simulink model "sampleModel931"  (R2021a)
settings: Solver=VariableStepAuto  StartTime=0.0  StopTime=10.0  RelTol=1e-3
undefined symbols (not defined in the file or in its folder): DiscIntNeverNeededParam, magnitude, Newton, Raphson
libraries: simulink x35, pid_lib x8
(part 1 of 2)
settings Model: Creator=user  LastModifiedBy=user

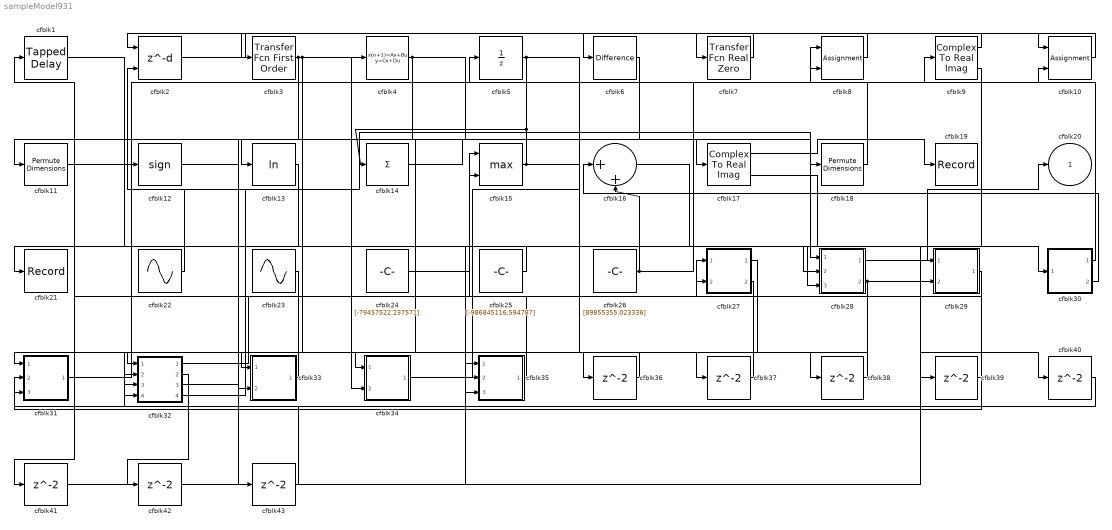
== system sampleModel931 ==
  cfblk1 : simulink/Discrete/Tapped Delay  vinit=0.0  samptime=-1  NumDelays=1  DelayOrder=Oldest  includeCurrent=off
  cfblk10 : Assignment  DiagnosticForDimensions=Warning  IndexOptions=Index vector (dialog)  Indices=1  OutputSizes=1
  cfblk11 : PermuteDimensions
  cfblk12 : Signum
  cfblk13 : Math  Operator=log  SaturateOnIntegerOverflow=on
  cfblk14 : Sum  Inputs=+
  cfblk15 : MinMax  Function=max  Inputs=2
  cfblk16 : Sum  Inputs=|++
  cfblk17 : ComplexToRealImag
  cfblk18 : PermuteDimensions
  cfblk19 : Record  FileSettingsInternal="{\"entries\":[{\"content\":{\"excelSettings\":{\"content\":{},\"type\":\"Streamout.ExcelSettings\"}},\"type\":\"Streamout.FileSettingStorage\",\"uuid\":\"344b2579-8096-44a0-829a-8fa8cea9bf3e\"}],\"packageUris\":[\"http://schema.mathworks.com/mf0/streamout_blocks/R2020a\"],\"version\":\"1.0\"}"  SignalsInternal="{\"entries\":[{\"content\":{\"signals\":[{\"content\":{\"blockPath\":[\"sampleModel931/cfblk19\"],\"channel\":[],\"dimensions\":[1],\"domain\":\"samplemodel931/cfblk19\",\"lineColor\":\"#a2142f\",\"plots\":[1],\"port\":1,\"sid\":[\"\"],\"signalID\":7177,\"signalName\":\"cfblk17:1\"},\"type\":\"RecordBlkView.Signal\",\"uuid\":\"202db960-daa0-4a0a-ad9f-c9ed2231518e\"}]},\"type\":\"RecordBlkView.InputSignals\",\"uuid\":\"c8fea5f5-595d-44bd-9296-e1420b6ba1ce\"}],\"packageUris\":[\"http://schema.mathworks.com/mf0/streamout_blocks/R2020a\"],\"version\":\"1.0\"}"  VisualizationBindings="{\"sparklinesplugin\":{\"info\":[{\"bindingParametersList\":[],\"subplotID\":1}]}}"
  cfblk2 : Delay  DelayLengthSource=Input port  SampleTime=1
      settings: InputPortMap=u0,p1
  cfblk21 : Record  FileSettingsInternal="{\"entries\":[{\"content\":{\"excelSettings\":{\"content\":{},\"type\":\"Streamout.ExcelSettings\"}},\"type\":\"Streamout.FileSettingStorage\",\"uuid\":\"47128032-d6b5-40ff-842c-bb4838ad83b6\"}],\"packageUris\":[\"http://schema.mathworks.com/mf0/streamout_blocks/R2020a\"],\"version\":\"1.0\"}"  SignalsInternal="{\"entries\":[{\"content\":{\"signals\":[{\"content\":{\"blockPath\":[\"sampleModel931/cfblk21\"],\"channel\":[],\"dimensions\":[1],\"domain\":\"samplemodel931/cfblk21\",\"lineColor\":\"#ff6929\",\"plots\":[1],\"port\":1,\"sid\":[\"\"],\"signalID\":7185,\"signalName\":\"cfblk25\"},\"type\":\"RecordBlkView.Signal\",\"uuid\":\"305fc408-6697-4ad2-987d-cf51be774916\"}]},\"type\":\"RecordBlkView.InputSignals\",\"uuid\":\"d64a9699-7d60-471f-aacd-da0b4468fcb5\"}],\"packageUris\":[\"http://schema.mathworks.com/mf0/streamout_blocks/R2020a\"],\"version\":\"1.0\"}"  VisualizationBindings="{\"sparklinesplugin\":{\"info\":[{\"bindingParametersList\":[],\"subplotID\":1}]}}"
  cfblk22 : Sin  Amplitude=[-979508255.020901]  Bias=[-315371967.281883]  SampleTime=0
  cfblk23 : Sin  Amplitude=[-6086076.617580]  Bias=[-663456107.750280]  SampleTime=0
  cfblk24 : Constant  Value=[-79457522.237571]  SampleTime=1
  cfblk25 : Constant  Value=[-986845116.594787]  SampleTime=1
  cfblk26 : Constant  Value=[89855355.023336]  SampleTime=1
  cfblk27 : Subsystem
  cfblk28 : Subsystem
  cfblk29 : Subsystem
  cfblk3 : simulink/Discrete/Transfer Fcn First Order  PoleZ=0.95  ICPrevOutput=0.0  DoSatur=off
  cfblk30 : Subsystem
  cfblk31 : Subsystem
  cfblk32 : Subsystem
  cfblk33 : Subsystem
  cfblk34 : Subsystem
  cfblk35 : Subsystem
  cfblk{36..43} (8 alike) : Delay  SampleTime=1
  cfblk4 : DiscreteStateSpace
  cfblk5 : UnitDelay  HasFrameUpgradeWarning=on
  cfblk6 : simulink/Discrete/Difference  ICPrevInput=0.0  OutMin=[]  OutMax=[]  OutDataTypeStr=Inherit: Inherit via back propagation  OutDataType=fixdt(1, 16)  OutScaling=2^-10  DoSatur=off
  cfblk7 : simulink/Discrete/Transfer Fcn Real Zero  ZeroZ=0.75  ICPrevInput=0.0  DoSatur=off
      settings: SourceProductBaseCode=SL
  cfblk8 : Assignment  DiagnosticForDimensions=Warning  IndexOptions=Index vector (dialog)  Indices=1  OutputSizes=1
  cfblk9 : ComplexToRealImag
  cfblk20 : Outport
  wires:
  cfblk2/1 -> cfblk10/1
  cfblk3/1 -> cfblk33/1(cfblk1), cfblk36/1, cfblk33/2(cfblk12)
  cfblk32/1(cfblk2) -> cfblk27/1(cfblk1)
  cfblk28/1(cfblk2) -> cfblk20/1
  cfblk35/1(cfblk2) -> cfblk15/1
  cfblk14/1 -> cfblk17/1
  cfblk11/1 -> cfblk28/1(cfblk1)
  cfblk5/1 -> cfblk14/1, cfblk34/1(cfblk1), cfblk28/3(cfblk14)
  cfblk4/1 -> cfblk11/1, cfblk18/1
  cfblk6/1 -> cfblk13/1
  cfblk8/1 -> cfblk2/1
  cfblk17/1 -> cfblk19/1
  cfblk25/1 -> cfblk21/1
  cfblk16/1 -> cfblk28/2(cfblk13)
  cfblk31/1(cfblk2) -> cfblk9/1
  cfblk33/1(cfblk2) -> cfblk32/1(cfblk1)
  cfblk18/1 -> cfblk8/1
  cfblk9/1 -> cfblk3/1
  cfblk22/1 -> cfblk2/2
  cfblk30/1(cfblk2) -> cfblk5/1
  cfblk30/2(cfblk8) -> cfblk16/1
  cfblk34/1(cfblk2) -> cfblk10/2
  cfblk29/1(cfblk2) -> cfblk31/2(cfblk13)
  cfblk32/4(cfblk16) -> cfblk4/1
  cfblk15/1 -> cfblk12/1, cfblk38/1
  cfblk24/1 -> cfblk15/2
  cfblk7/1 -> cfblk6/1
  cfblk26/1 -> cfblk8/2, cfblk16/2
  cfblk1/1 -> cfblk29/2(cfblk12)
  cfblk10/1 -> cfblk7/1
  cfblk28/2(cfblk15) -> cfblk34/2(cfblk7), cfblk40/1
  cfblk9/2 -> cfblk35/2(cfblk16)
  cfblk12/1 -> cfblk30/1(cfblk1)
  cfblk23/1 -> cfblk32/4(cfblk13)
  cfblk27/2(cfblk7) -> cfblk35/3(cfblk17)
  cfblk36/1 -> cfblk31/1(cfblk1)
  cfblk27/1(cfblk2) -> cfblk37/1
  cfblk37/1 -> cfblk1/1
  cfblk38/1 -> cfblk32/2(cfblk11)
  cfblk17/2 -> cfblk39/1
  cfblk39/1 -> cfblk27/2(cfblk6)
  cfblk40/1 -> cfblk32/3(cfblk12)
  cfblk13/1 -> cfblk41/1
  cfblk41/1 -> cfblk35/1(cfblk1)
  cfblk32/2(cfblk14) -> cfblk42/1
  cfblk42/1 -> cfblk29/1(cfblk1)
  cfblk32/3(cfblk15) -> cfblk43/1
  cfblk43/1 -> cfblk31/3(cfblk14)

== system sampleModel931/cfblk27 ==
  cfblk1 : Inport
  cfblk6 : Inport  Port=2
  cfblk3 : Constant  Value=[-684045986.620494]  SampleTime=1
  cfblk4 : Subsystem
  cfblk5 : Subsystem
  cfblk2 : Outport
  cfblk7 : Outport  Port=2
  wires:
  cfblk5/1(cfblk2) -> cfblk7/1
  cfblk6/1 -> cfblk5/1(cfblk1)
  cfblk1/1 -> cfblk5/2(cfblk13)
  cfblk3/1 -> cfblk2/1
  cfblk5/2(cfblk14) -> cfblk4/1(cfblk1)

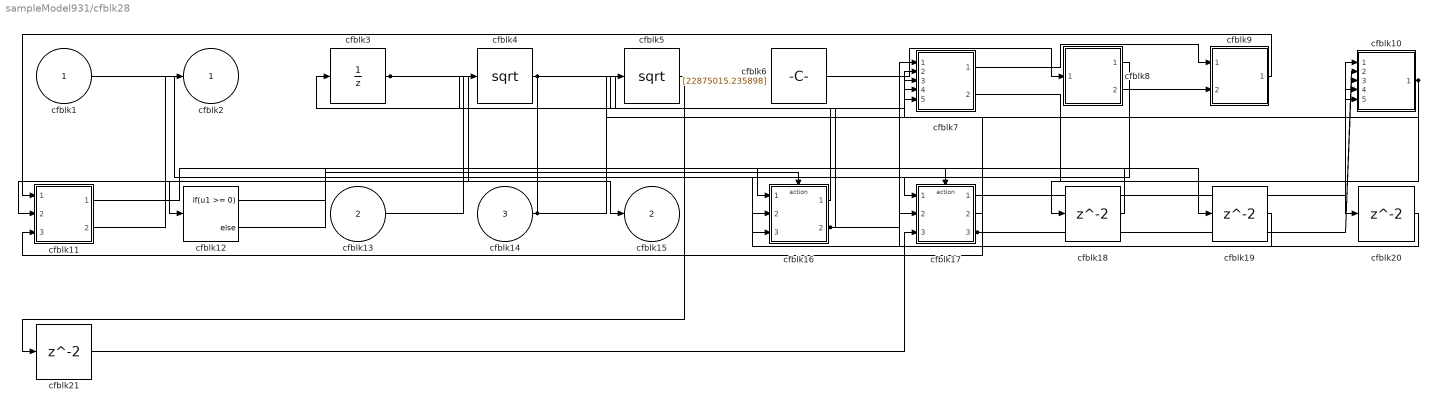
== system sampleModel931/cfblk28 ==
  cfblk1 : Inport
  cfblk13 : Inport  Port=2
  cfblk14 : Inport  Port=3
  cfblk10 : Subsystem
  cfblk11 : Subsystem
  cfblk12 : If  IfExpression=u1 >= 0  SampleTime=1
  cfblk16 : Subsystem  TreatAsAtomicUnit=on
  cfblk17 : Subsystem  TreatAsAtomicUnit=on
  cfblk{18..21} (4 alike) : Delay  SampleTime=1
  cfblk3 : UnitDelay  HasFrameUpgradeWarning=on
  cfblk4 : Sqrt  SaturateOnIntegerOverflow=on
  cfblk5 : Sqrt  SaturateOnIntegerOverflow=on
  cfblk6 : Constant  Value=[22875015.235898]  SampleTime=1
  cfblk7 : Subsystem
  cfblk8 : Subsystem
  cfblk9 : Subsystem
  cfblk2 : Outport
  cfblk15 : Outport  Port=2
  wires:
  cfblk17/1(cfblk2) -> cfblk10/1(cfblk1)
  cfblk1/1 -> cfblk17/1(cfblk1)
  cfblk7/1(cfblk2) -> cfblk9/1(cfblk1)
  cfblk10/1(cfblk2) -> cfblk7/4(cfblk12), cfblk18/1
  cfblk8/1(cfblk2) -> cfblk16/3(cfblk14)
  cfblk3/1 -> cfblk15/1, cfblk7/5(cfblk13)
  cfblk14/1 -> cfblk12/1, cfblk10/4(cfblk15)
  cfblk8/2(cfblk8) -> cfblk9/2(cfblk15)
  cfblk13/1 -> cfblk4/1
  cfblk16/1(cfblk2) -> cfblk3/1
  cfblk9/1(cfblk2) -> cfblk11/1(cfblk1)
  cfblk11/2(cfblk15) -> cfblk2/1
  cfblk4/1 -> cfblk11/2(cfblk13), cfblk7/3(cfblk11), cfblk10/5(cfblk16)
  cfblk6/1 -> cfblk8/1(cfblk1)
  cfblk16/2(cfblk15) -> cfblk7/1(cfblk1), cfblk5/1
  cfblk17/2(cfblk13) -> cfblk11/3(cfblk14)
  cfblk17/3(cfblk14) -> cfblk7/2(cfblk10), cfblk10/2(cfblk13), cfblk10/3(cfblk14)
  cfblk12/1 -> cfblk16/Action
  cfblk12/2 -> cfblk17/Action
  cfblk18/1 -> cfblk16/1(cfblk1)
  cfblk11/1(cfblk2) -> cfblk19/1
  cfblk19/1 -> cfblk17/2(cfblk11)
  cfblk7/2(cfblk14) -> cfblk20/1
  cfblk20/1 -> cfblk16/2(cfblk13)
  cfblk5/1 -> cfblk21/1
  cfblk21/1 -> cfblk17/3(cfblk12)

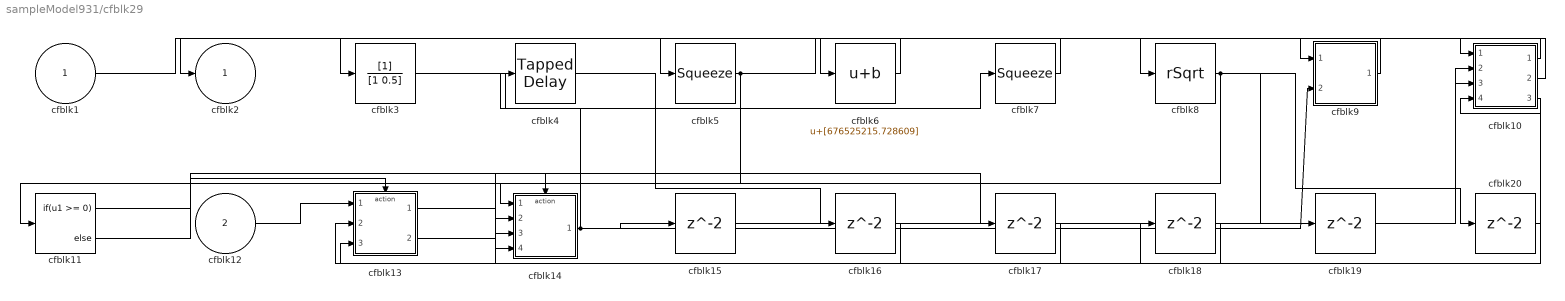
== system sampleModel931/cfblk29 ==
  cfblk1 : Inport
  cfblk12 : Inport  Port=2
  cfblk10 : Subsystem
  cfblk11 : If  IfExpression=u1 >= 0  SampleTime=1
  cfblk13 : Subsystem  TreatAsAtomicUnit=on
  cfblk14 : Subsystem  TreatAsAtomicUnit=on
  cfblk{15..20} (6 alike) : Delay  SampleTime=1
  cfblk3 : DiscreteFilter  SampleTime=1
  cfblk4 : simulink/Discrete/Tapped Delay  vinit=0.0  samptime=-1  NumDelays=1  DelayOrder=Oldest  includeCurrent=off
  cfblk5 : Squeeze
  cfblk6 : Bias  Bias=[676525215.728609]
  cfblk7 : Squeeze
  cfblk8 : Sqrt  Operator=rSqrt  AlgorithmType=Newton-Raphson  SaturateOnIntegerOverflow=on
  cfblk9 : Subsystem
  cfblk2 : Outport
  wires:
  cfblk9/1(cfblk2) -> cfblk3/1
  cfblk3/1 -> cfblk7/1
  cfblk6/1 -> cfblk2/1
  cfblk7/1 -> cfblk6/1
  cfblk12/1 -> cfblk13/1(cfblk1)
  cfblk1/1 -> cfblk5/1
  cfblk8/1 -> cfblk14/1(cfblk1), cfblk19/1, cfblk20/1
  cfblk5/1 -> cfblk10/1(cfblk1), cfblk11/1, cfblk14/4(cfblk14)
  cfblk10/1(cfblk2) -> cfblk8/1
  cfblk14/1(cfblk2) -> cfblk9/2(cfblk8), cfblk4/1, cfblk15/1
  cfblk10/2(cfblk9) -> cfblk9/1(cfblk1)
  cfblk10/3(cfblk10) -> cfblk13/3(cfblk16)
  cfblk11/1 -> cfblk13/Action
  cfblk11/2 -> cfblk14/Action
  cfblk15/1 -> cfblk10/2(cfblk6)
  cfblk4/1 -> cfblk16/1
  cfblk16/1 -> cfblk13/2(cfblk15)
  cfblk13/1(cfblk2) -> cfblk17/1
  cfblk17/1 -> cfblk14/2(cfblk12)
  cfblk13/2(cfblk17) -> cfblk18/1
  cfblk18/1 -> cfblk14/3(cfblk13)
  cfblk19/1 -> cfblk10/3(cfblk7)
  cfblk20/1 -> cfblk10/4(cfblk8)

== system sampleModel931/cfblk30 ==
  cfblk1 : Inport
  cfblk3 : DiscreteFir  SampleTime=1
  cfblk4 : DiscreteStateSpace
  cfblk5 : Product
  cfblk6 : Product
  cfblk7 : Constant  Value=[840177180.209382]  SampleTime=1
  cfblk2 : Outport
  cfblk8 : Outport  Port=2
  wires:
  cfblk7/1 -> cfblk6/1
  cfblk5/1 -> cfblk3/1, cfblk4/1
  cfblk3/1 -> cfblk6/2
  cfblk4/1 -> cfblk8/1
  cfblk1/1 -> cfblk5/1, cfblk5/2
  cfblk6/1 -> cfblk2/1

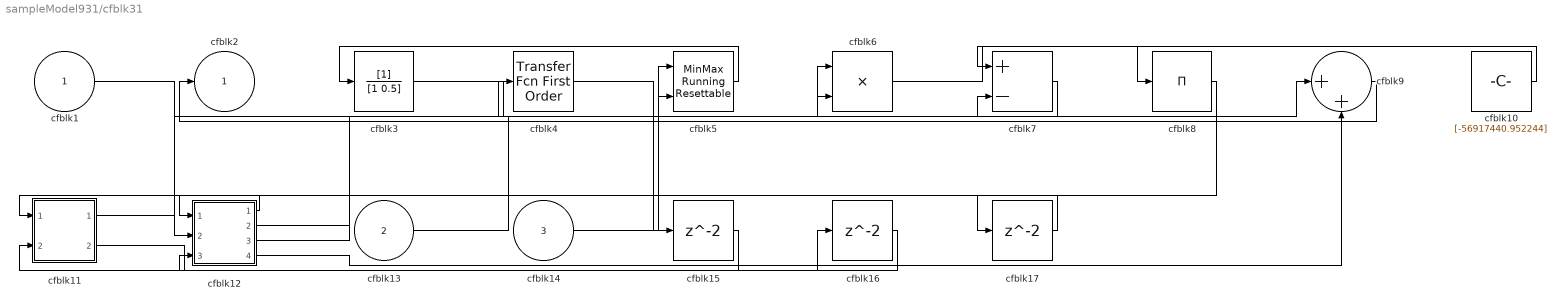
== system sampleModel931/cfblk31 ==
  cfblk1 : Inport
  cfblk13 : Inport  Port=2
  cfblk14 : Inport  Port=3
  cfblk10 : Constant  Value=[-56917440.952244]  SampleTime=1
  cfblk11 : Subsystem
  cfblk12 : Subsystem
  cfblk15 : Delay  SampleTime=1
  cfblk16 : Delay  SampleTime=1
  cfblk17 : Delay  SampleTime=1
  cfblk3 : DiscreteFilter  SampleTime=1
  cfblk4 : simulink/Discrete/Transfer Fcn First Order  PoleZ=0.95  ICPrevOutput=0.0  DoSatur=off
  cfblk5 : simulink/Math Operations/MinMax Running Resettable  Function=min  vinit=0.0
  cfblk6 : Product
  cfblk7 : Sum  Inputs=+-
  cfblk8 : Product  Inputs=*
  cfblk9 : Sum  Inputs=|++
  cfblk2 : Outport
  wires:
  cfblk6/1 -> cfblk8/1
  cfblk9/1 -> cfblk2/1
  cfblk5/1 -> cfblk3/1
  cfblk3/1 -> cfblk6/1
  cfblk10/1 -> cfblk7/1
  cfblk7/1 -> cfblk6/2
  cfblk11/1(cfblk2) -> cfblk4/1
  cfblk13/1 -> cfblk9/1
  cfblk12/1(cfblk2) -> cfblk11/1(cfblk1)
  cfblk1/1 -> cfblk12/2(cfblk10)
  cfblk12/2(cfblk12) -> cfblk7/2
  cfblk12/3(cfblk13) -> cfblk5/1
  cfblk14/1 -> cfblk5/2
  cfblk12/4(cfblk14) -> cfblk9/2
  cfblk4/1 -> cfblk15/1
  cfblk15/1 -> cfblk11/2(cfblk6)
  cfblk11/2(cfblk7) -> cfblk16/1
  cfblk16/1 -> cfblk12/3(cfblk11)
  cfblk8/1 -> cfblk17/1
  cfblk17/1 -> cfblk12/1(cfblk1)

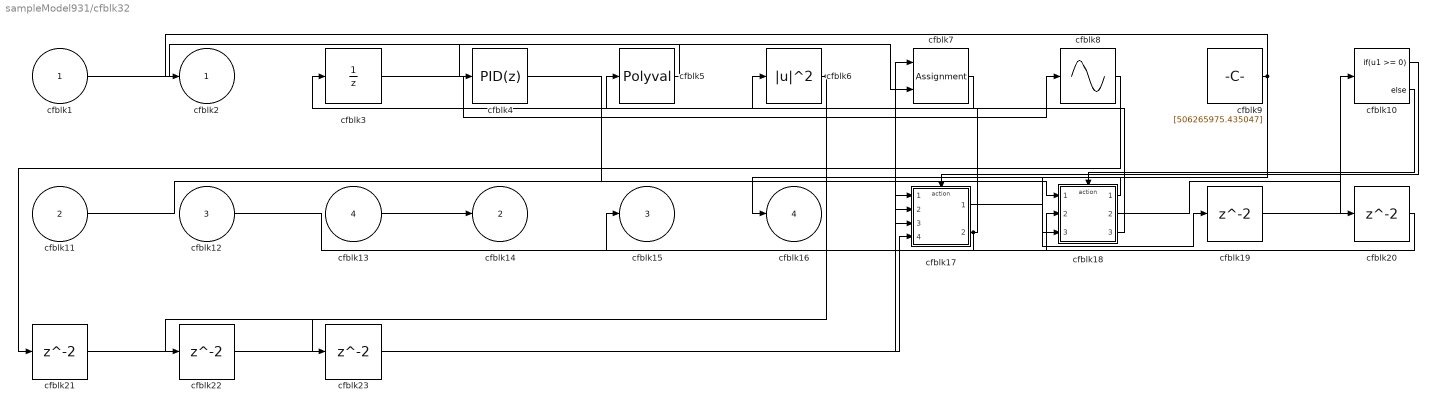
== system sampleModel931/cfblk32 ==
  cfblk1 : Inport
  cfblk11 : Inport  Port=2
  cfblk12 : Inport  Port=3
  cfblk13 : Inport  Port=4
  cfblk10 : If  IfExpression=u1 >= 0  SampleTime=1
  cfblk17 : Subsystem  TreatAsAtomicUnit=on
  cfblk18 : Subsystem  TreatAsAtomicUnit=on
  cfblk{19..23} (5 alike) : Delay  SampleTime=1
  cfblk3 : UnitDelay  HasFrameUpgradeWarning=on
  cfblk4 : pid_lib/PID Controller  Controller=PID  Form=Parallel  TimeDomain=Discrete-time  UseExternalTs=off  SampleTime=1  IntegratorMethod=Forward Euler  FilterMethod=Forward Euler  ControllerParametersSource=internal  P=1  I=1  D=0  UseFilter=on  N=100  TunerSelectOption=Transfer Function Based (PID Tuner App)  InitialConditionSource=internal  InitialConditionForIntegrator=0  InitialConditionForFilter=0  DifferentiatorICPrevScaledInput=0  ExternalReset=none  TrackingMode=off  Kt=1  LimitOutput=off  SatLimitsSource=internal  UpperSaturationLimit=inf  LowerSaturationLimit=-inf  LinearizeAsGain=off  AntiWindupMode=none  Kb=1  POutMin=[]  POutMax=[]  IOutMin=[]  IOutMax=[]  DOutMin=[]  DOutMax=[]  NOutMin=[]  NOutMax=[]  SumOutMin=[]  SumOutMax=[]  SaturationOutMin=[]  SaturationOutMax=[]  PParamMin=[]  PParamMax=[]  IParamMin=[]  IParamMax=[]  DParamMin=[]  DParamMax=[]  NParamMin=[]  NParamMax=[]  KbParamMin=[]  KbParamMax=[]  KtParamMin=[]  KtParamMax=[]  KbOutMin=[]  KbOutMax=[]  KtOutMin=[]  KtOutMax=[]  IntegratorOutMin=[]  IntegratorOutMax=[]  FilterOutMin=[]  FilterOutMax=[]  SumI1OutMin=[]  SumI1OutMax=[]  SumI2OutMin=[]  SumI2OutMax=[]  SumI3OutMin=[]  SumI3OutMax=[]  SumI4OutMin=[]  SumI4OutMax=[]  SumDOutMin=[]  SumDOutMax=[]  DifferentiatorOutMin=[]  DifferentiatorOutMax=[]  FilterDiffOutCoefMin=[]  FilterDiffOutCoefMax=[]  ReciprocalOutMin=[]  ReciprocalOutMax=[]  SumDenOutMin=[]  SumDenOutMax=[]  SumNumOutMin=[]  SumNumOutMax=[]  DivideOutMin=[]  DivideOutMax=[]  UdiffTsProdOutMin=[]  UdiffTsProdOutMax=[]  NTsProdOutMin=[]  NTsProdOutMax=[]  UintegralTsProdOutMin=[]  UintegralTsProdOutMax=[]  UngainTsProdOutMin=[]  UngainTsProdOutMax=[]  IntegratorContinuousStateAttributes=''  IntegratorStateMustResolveToSignalObject=off  IntegratorRTWStateStorageClass=Auto  FilterContinuousStateAttributes=''  FilterStateMustResolveToSignalObject=off  FilterRTWStateStorageClass=Auto  ParallelPVariant=InternalParameters  IdealPVariant=Disabled  IVariant=InternalParameters  DVariant=InternalParameters  IntegratorVariant=Discrete  SatVariant=Disabled  AWVariant=Passthrough  PCopyVariant=Disabled  TRVariant=Disabled  FdbkBlocksVariant=Forward  IdealPFdbkVariant=Disabled  SatFdbkVariant=Disabled  DerivativeFilterVariant=ForwardEulerFilter  NVariant=InternalParameters  NCopyVariant=Disabled  FilterICVariant=InternalICsFilter  IntegratorICVariant=InternalICs  ExternalResetVariant=Disabled  TRSumVariant=Passthrough  SumFdbkVariant=Disabled  SumVariant=Sum_PID  TsampFilterVariant=InternalTs  TsampNgainVariant=Passthrough  TsampIntegralVariant=Passthrough  ExternalSaturationOutDataTypeStr=Inherit: Same as second input
  cfblk5 : Polyval  Coefs=[ +2.081618890e-019, -1.441693666e-014, +4.719686976e-010, -8.536869453e-006, +1.621573104e-001, -8.087801117e+001 ]
  cfblk6 : Math  Operator=magnitude^2  SaturateOnIntegerOverflow=on
  cfblk7 : Assignment  DiagnosticForDimensions=Warning  IndexOptions=Index vector (dialog)  Indices=1  OutputSizes=1
  cfblk8 : Sin  TimeSource=Use external signal  SampleTime=0
  cfblk9 : Constant  Value=[506265975.435047]  SampleTime=1
  cfblk2 : Outport
  cfblk14 : Outport  Port=2
  cfblk15 : Outport  Port=3
  cfblk16 : Outport  Port=4
  wires:
  cfblk11/1 -> cfblk18/1(cfblk1)
  cfblk13/1 -> cfblk14/1
  cfblk12/1 -> cfblk18/2(cfblk9)
  cfblk7/1 -> cfblk5/1
  cfblk18/1(cfblk2) -> cfblk16/1
  cfblk1/1 -> cfblk7/2
  cfblk9/1 -> cfblk2/1, cfblk18/3(cfblk10)
  cfblk3/1 -> cfblk8/1
  cfblk6/1 -> cfblk22/1, cfblk23/1
  cfblk17/2(cfblk17) -> cfblk6/1, cfblk15/1
  cfblk18/3(cfblk12) -> cfblk3/1
  cfblk5/1 -> cfblk4/1
  cfblk4/1 -> cfblk17/3(cfblk15)
  cfblk10/1 -> cfblk17/Action
  cfblk10/2 -> cfblk18/Action
  cfblk17/1(cfblk2) -> cfblk19/1
  cfblk19/1 -> cfblk10/1
  cfblk18/2(cfblk11) -> cfblk20/1
  cfblk20/1 -> cfblk17/2(cfblk14)
  cfblk8/1 -> cfblk21/1
  cfblk21/1 -> cfblk7/1
  cfblk22/1 -> cfblk17/1(cfblk1)
  cfblk23/1 -> cfblk17/4(cfblk16)

== system sampleModel931/cfblk33 ==
  cfblk1 : Inport
  cfblk12 : Inport  Port=2
  cfblk10 : Subsystem
  cfblk11 : Subsystem
  cfblk13 : Delay  SampleTime=1
  cfblk14 : Delay  SampleTime=1
  cfblk3 : DiscreteTransferFcn  SampleTime=1
  cfblk4 : pid_lib/PID Controller  Controller=PID  Form=Parallel  TimeDomain=Discrete-time  UseExternalTs=off  SampleTime=1  IntegratorMethod=Forward Euler  FilterMethod=Forward Euler  ControllerParametersSource=internal  P=1  I=1  D=0  UseFilter=on  N=100  TunerSelectOption=Transfer Function Based (PID Tuner App)  InitialConditionSource=internal  InitialConditionForIntegrator=0  InitialConditionForFilter=0  DifferentiatorICPrevScaledInput=0  ExternalReset=none  TrackingMode=off  Kt=1  LimitOutput=off  SatLimitsSource=internal  UpperSaturationLimit=inf  LowerSaturationLimit=-inf  LinearizeAsGain=off  AntiWindupMode=none  Kb=1  POutMin=[]  POutMax=[]  IOutMin=[]  IOutMax=[]  DOutMin=[]  DOutMax=[]  NOutMin=[]  NOutMax=[]  SumOutMin=[]  SumOutMax=[]  SaturationOutMin=[]  SaturationOutMax=[]  PParamMin=[]  PParamMax=[]  IParamMin=[]  IParamMax=[]  DParamMin=[]  DParamMax=[]  NParamMin=[]  NParamMax=[]  KbParamMin=[]  KbParamMax=[]  KtParamMin=[]  KtParamMax=[]  KbOutMin=[]  KbOutMax=[]  KtOutMin=[]  KtOutMax=[]  IntegratorOutMin=[]  IntegratorOutMax=[]  FilterOutMin=[]  FilterOutMax=[]  SumI1OutMin=[]  SumI1OutMax=[]  SumI2OutMin=[]  SumI2OutMax=[]  SumI3OutMin=[]  SumI3OutMax=[]  SumI4OutMin=[]  SumI4OutMax=[]  SumDOutMin=[]  SumDOutMax=[]  DifferentiatorOutMin=[]  DifferentiatorOutMax=[]  FilterDiffOutCoefMin=[]  FilterDiffOutCoefMax=[]  ReciprocalOutMin=[]  ReciprocalOutMax=[]  SumDenOutMin=[]  SumDenOutMax=[]  SumNumOutMin=[]  SumNumOutMax=[]  DivideOutMin=[]  DivideOutMax=[]  UdiffTsProdOutMin=[]  UdiffTsProdOutMax=[]  NTsProdOutMin=[]  NTsProdOutMax=[]  UintegralTsProdOutMin=[]  UintegralTsProdOutMax=[]  UngainTsProdOutMin=[]  UngainTsProdOutMax=[]  IntegratorContinuousStateAttributes=''  IntegratorStateMustResolveToSignalObject=off  IntegratorRTWStateStorageClass=Auto  FilterContinuousStateAttributes=''  FilterStateMustResolveToSignalObject=off  FilterRTWStateStorageClass=Auto  ParallelPVariant=InternalParameters  IdealPVariant=Disabled  IVariant=InternalParameters  DVariant=InternalParameters  IntegratorVariant=Discrete  SatVariant=Disabled  AWVariant=Passthrough  PCopyVariant=Disabled  TRVariant=Disabled  FdbkBlocksVariant=Forward  IdealPFdbkVariant=Disabled  SatFdbkVariant=Disabled  DerivativeFilterVariant=ForwardEulerFilter  NVariant=InternalParameters  NCopyVariant=Disabled  FilterICVariant=InternalICsFilter  IntegratorICVariant=InternalICs  ExternalResetVariant=Disabled  TRSumVariant=Passthrough  SumFdbkVariant=Disabled  SumVariant=Sum_PID  TsampFilterVariant=InternalTs  TsampNgainVariant=Passthrough  TsampIntegralVariant=Passthrough  ExternalSaturationOutDataTypeStr=Inherit: Same as second input
  cfblk5 : DiscreteFilter  SampleTime=1
  cfblk6 : UnaryMinus
  cfblk7 : Sin  TimeSource=Use external signal  SampleTime=0
  cfblk8 : Constant  Value=[249511604.295166]  SampleTime=1
  cfblk9 : Subsystem
  cfblk2 : Outport
  wires:
  cfblk10/1(cfblk2) -> cfblk4/1
  cfblk8/1 -> cfblk5/1
  cfblk5/1 -> cfblk3/1
  cfblk1/1 -> cfblk6/1
  cfblk4/1 -> cfblk13/1, cfblk14/1
  cfblk6/1 -> cfblk7/1, cfblk9/2(cfblk5)
  cfblk3/1 -> cfblk10/2(cfblk7)
  cfblk10/2(cfblk9) -> cfblk2/1
  cfblk12/1 -> cfblk11/1(cfblk1), cfblk9/3(cfblk6)
  cfblk7/1 -> cfblk11/2(cfblk9)
  cfblk11/1(cfblk2) -> cfblk9/1(cfblk1)
  cfblk9/1(cfblk2) -> cfblk10/3(cfblk8)
  cfblk13/1 -> cfblk10/1(cfblk1)
  cfblk14/1 -> cfblk9/4(cfblk7)

== system sampleModel931/cfblk34 ==
  cfblk1 : Inport
  cfblk7 : Inport  Port=2
  cfblk3 : DiscreteIntegrator  ICPrevOutput=DiscIntNeverNeededParam  ICPrevScaledInput=DiscIntNeverNeededParam
  cfblk4 : Assignment  DiagnosticForDimensions=Warning  IndexOptions=Index vector (dialog)  Indices=1  OutputSizes=1
  cfblk5 : Gain  Gain=[-574459450.541331]
  cfblk6 : Constant  Value=[554501118.306872]  SampleTime=1
  cfblk8 : Delay  SampleTime=1
  cfblk2 : Outport
  wires:
  cfblk6/1 -> cfblk2/1
  cfblk3/1 -> cfblk4/1
  cfblk1/1 -> cfblk5/1
  cfblk7/1 -> cfblk4/2
  cfblk4/1 -> cfblk8/1
  cfblk8/1 -> cfblk3/1

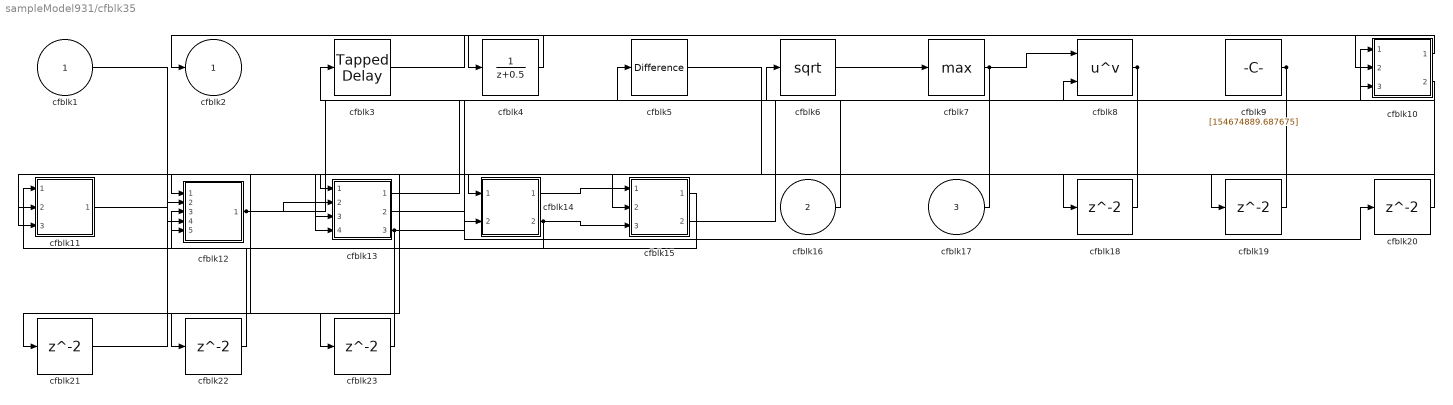
== system sampleModel931/cfblk35 ==
  cfblk1 : Inport
  cfblk16 : Inport  Port=2
  cfblk17 : Inport  Port=3
  cfblk10 : Subsystem
  cfblk11 : Subsystem
  cfblk12 : Subsystem
  cfblk13 : Subsystem
  cfblk14 : Subsystem
  cfblk15 : Subsystem
  cfblk{18..23} (6 alike) : Delay  SampleTime=1
  cfblk3 : simulink/Discrete/Tapped Delay  vinit=0.0  samptime=-1  NumDelays=1  DelayOrder=Oldest  includeCurrent=off
  cfblk4 : DiscreteTransferFcn  SampleTime=1
  cfblk5 : simulink/Discrete/Difference  ICPrevInput=0.0  OutMin=[]  OutMax=[]  OutDataTypeStr=Inherit: Inherit via back propagation  OutDataType=fixdt(1, 16)  OutScaling=2^-10  DoSatur=off
  cfblk6 : Sqrt  SaturateOnIntegerOverflow=on
  cfblk7 : MinMax  Function=max
  cfblk8 : Math  Operator=pow  SaturateOnIntegerOverflow=on
  cfblk9 : Constant  Value=[154674889.687675]  SampleTime=1
  cfblk2 : Outport
  wires:
  cfblk7/1 -> cfblk8/1, cfblk23/1
  cfblk9/1 -> cfblk14/1(cfblk1), cfblk13/4(cfblk12)
  cfblk15/1(cfblk2) -> cfblk11/1(cfblk1)
  cfblk4/1 -> cfblk2/1
  cfblk13/1(cfblk2) -> cfblk5/1
  cfblk6/1 -> cfblk7/1
  cfblk12/1(cfblk2) -> cfblk6/1, cfblk13/2(cfblk10)
  cfblk16/1 -> cfblk3/1
  cfblk10/1(cfblk2) -> cfblk4/1
  cfblk14/1(cfblk2) -> cfblk15/1(cfblk1)
  cfblk15/2(cfblk15) -> cfblk10/1(cfblk1)
  cfblk10/2(cfblk11) -> cfblk11/2(cfblk12)
  cfblk8/1 -> cfblk11/3(cfblk13), cfblk13/3(cfblk11), cfblk22/1
  cfblk14/2(cfblk7) -> cfblk15/3(cfblk14), cfblk12/3(cfblk9)
  cfblk3/1 -> cfblk10/2(cfblk9)
  cfblk1/1 -> cfblk14/2(cfblk6)
  cfblk13/3(cfblk14) -> cfblk10/3(cfblk10), cfblk21/1
  cfblk17/1 -> cfblk12/1(cfblk1)
  cfblk11/1(cfblk2) -> cfblk18/1
  cfblk18/1 -> cfblk15/2(cfblk13)
  cfblk5/1 -> cfblk19/1
  cfblk19/1 -> cfblk13/1(cfblk1)
  cfblk13/2(cfblk13) -> cfblk20/1
  cfblk20/1 -> cfblk8/2
  cfblk21/1 -> cfblk12/4(cfblk10)
  cfblk22/1 -> cfblk12/5(cfblk11)
  cfblk23/1 -> cfblk12/2(cfblk8)

== system sampleModel931/cfblk27/cfblk4 ==
  cfblk1 : Inport
  cfblk10 : Constant  Value=[-976092899.684537]  SampleTime=1
  cfblk16 : Delay  SampleTime=1
  cfblk3 : Delay  DelayLengthSource=Input port  SampleTime=1
      settings: InputPortMap=u0,p1
  cfblk4 : DiscreteFir  SampleTime=1
  cfblk5 : DiscreteIntegrator  ICPrevOutput=DiscIntNeverNeededParam  ICPrevScaledInput=DiscIntNeverNeededParam
  cfblk6 : Sin  TimeSource=Use external signal  SampleTime=0
  cfblk7 : Trigonometry
  cfblk8 : Trigonometry
  cfblk9 : Abs
  cfblk2 : Outport
  cfblk11 : Outport  Port=2
  cfblk12 : Outport  Port=3
  cfblk13 : Outport  Port=4
  cfblk14 : Outport  Port=5
  cfblk15 : Outport  Port=6
  wires:
  cfblk9/1 -> cfblk13/1, cfblk12/1
  cfblk5/1 -> cfblk2/1, cfblk7/1, cfblk4/1
  cfblk8/1 -> cfblk5/1
  cfblk4/1 -> cfblk6/1
  cfblk10/1 -> cfblk11/1, cfblk3/2
  cfblk1/1 -> cfblk9/1
  cfblk3/1 -> cfblk8/1
  cfblk6/1 -> cfblk14/1, cfblk16/1
  cfblk7/1 -> cfblk15/1
  cfblk16/1 -> cfblk3/1

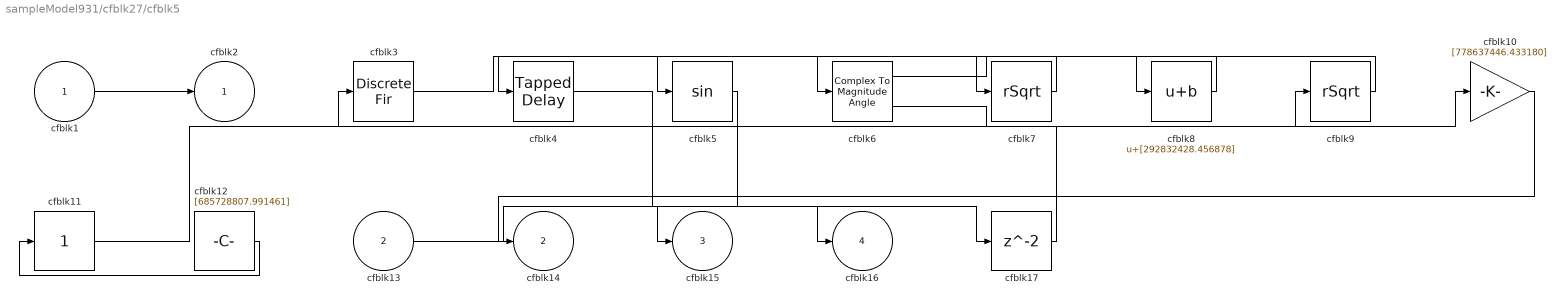
== system sampleModel931/cfblk27/cfblk5 ==
  cfblk1 : Inport
  cfblk13 : Inport  Port=2
  cfblk10 : Gain  Gain=[778637446.433180]
  cfblk11 : simulink/Math Operations/Slider Gain  gain=1  low=0  high=2
  cfblk12 : Constant  Value=[685728807.991461]  SampleTime=1
  cfblk17 : Delay  SampleTime=1
  cfblk3 : DiscreteFir  SampleTime=1
  cfblk4 : simulink/Discrete/Tapped Delay  vinit=0.0  samptime=-1  NumDelays=1  DelayOrder=Oldest  includeCurrent=off
  cfblk5 : Trigonometry
  cfblk6 : ComplexToMagnitudeAngle
  cfblk7 : Sqrt  Operator=rSqrt  AlgorithmType=Newton-Raphson  SaturateOnIntegerOverflow=on
  cfblk8 : Bias  Bias=[292832428.456878]
  cfblk9 : Sqrt  Operator=rSqrt  AlgorithmType=Newton-Raphson  SaturateOnIntegerOverflow=on
  cfblk2 : Outport
  cfblk14 : Outport  Port=2
  cfblk15 : Outport  Port=3
  cfblk16 : Outport  Port=4
  wires:
  cfblk11/1 -> cfblk9/1
  cfblk12/1 -> cfblk11/1
  cfblk13/1 -> cfblk16/1
  cfblk8/1 -> cfblk7/1
  cfblk7/1 -> cfblk4/1
  cfblk1/1 -> cfblk2/1
  cfblk10/1 -> cfblk14/1
  cfblk9/1 -> cfblk5/1
  cfblk5/1 -> cfblk15/1
  cfblk3/1 -> cfblk6/1
  cfblk6/1 -> cfblk8/1
  cfblk6/2 -> cfblk10/1
  cfblk4/1 -> cfblk17/1
  cfblk17/1 -> cfblk3/1

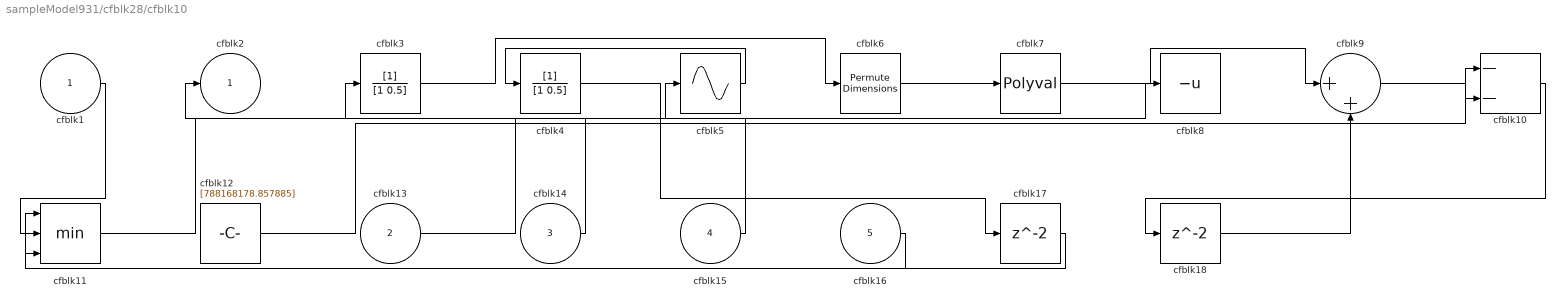
== system sampleModel931/cfblk28/cfblk10 ==
  cfblk1 : Inport
  cfblk13 : Inport  Port=2
  cfblk14 : Inport  Port=3
  cfblk15 : Inport  Port=4
  cfblk16 : Inport  Port=5
  cfblk10 : Sum  Inputs=--
  cfblk11 : MinMax  Inputs=3
  cfblk12 : Constant  Value=[788168178.857885]  SampleTime=1
  cfblk17 : Delay  SampleTime=1
  cfblk18 : Delay  SampleTime=1
  cfblk3 : DiscreteFilter  SampleTime=1
  cfblk4 : DiscreteFilter  SampleTime=1
  cfblk5 : Sin  TimeSource=Use external signal  SampleTime=0
  cfblk6 : PermuteDimensions
  cfblk7 : Polyval  Coefs=[ +2.081618890e-019, -1.441693666e-014, +4.719686976e-010, -8.536869453e-006, +1.621573104e-001, -8.087801117e+001 ]
  cfblk8 : UnaryMinus
  cfblk9 : Sum  Inputs=|++
  cfblk2 : Outport
  wires:
  cfblk6/1 -> cfblk7/1
  cfblk12/1 -> cfblk10/1
  cfblk11/1 -> cfblk5/1
  cfblk14/1 -> cfblk3/1
  cfblk15/1 -> cfblk2/1
  cfblk5/1 -> cfblk4/1
  cfblk7/1 -> cfblk9/1
  cfblk16/1 -> cfblk11/1
  cfblk1/1 -> cfblk11/2
  cfblk13/1 -> cfblk8/1
  cfblk3/1 -> cfblk6/1
  cfblk9/1 -> cfblk10/2
  cfblk4/1 -> cfblk17/1
  cfblk17/1 -> cfblk11/3
  cfblk10/1 -> cfblk18/1
  cfblk18/1 -> cfblk9/2

== system sampleModel931/cfblk28/cfblk11 ==
  cfblk1 : Inport
  cfblk13 : Inport  Port=2
  cfblk14 : Inport  Port=3
  cfblk10 : Constant  Value=[318220619.470984]  SampleTime=1
  cfblk11 : Constant  Value=[-256392654.534912]  SampleTime=1
  cfblk12 : Constant  Value=[-197992999.193617]  SampleTime=1
  cfblk16 : Delay  SampleTime=1
  cfblk3 : DiscreteFilter  SampleTime=1
  cfblk4 : simulink/Discrete/Difference  ICPrevInput=0.0  OutMin=[]  OutMax=[]  OutDataTypeStr=Inherit: Inherit via back propagation  OutDataType=fixdt(1, 16)  OutScaling=2^-10  DoSatur=off
  cfblk5 : simulink/Discrete/Transfer Fcn Lead or Lag  PoleZ=0.95  ZeroZ=0.75  ICPrevOutput=0.0  ICPrevInput=0.0  DoSatur=off
      settings: SourceProductBaseCode=SL
  cfblk6 : pid_lib/PID Controller (2DOF)  Controller=PID  Form=Parallel  TimeDomain=Discrete-time  UseExternalTs=off  SampleTime=1  IntegratorMethod=Forward Euler  FilterMethod=Forward Euler  ControllerParametersSource=internal  P=1  I=1  D=0  UseFilter=on  N=100  b=1  c=1  TunerSelectOption=Transfer Function Based (PID Tuner App)  InitialConditionSource=internal  InitialConditionForIntegrator=0  InitialConditionForFilter=0  DifferentiatorICPrevScaledInput=0  ExternalReset=none  TrackingMode=off  Kt=1  LimitOutput=off  SatLimitsSource=internal  UpperSaturationLimit=inf  LowerSaturationLimit=-inf  LinearizeAsGain=off  AntiWindupMode=none  Kb=1  POutMin=[]  POutMax=[]  IOutMin=[]  IOutMax=[]  DOutMin=[]  DOutMax=[]  NOutMin=[]  NOutMax=[]  bOutMin=[]  bOutMax=[]  cOutMin=[]  cOutMax=[]  SumOutMin=[]  SumOutMax=[]  SaturationOutMin=[]  SaturationOutMax=[]  PParamMin=[]  PParamMax=[]  IParamMin=[]  IParamMax=[]  DParamMin=[]  DParamMax=[]  NParamMin=[]  NParamMax=[]  bParamMin=[]  bParamMax=[]  cParamMin=[]  cParamMax=[]  KbParamMin=[]  KbParamMax=[]  KtParamMin=[]  KtParamMax=[]  KbOutMin=[]  KbOutMax=[]  KtOutMin=[]  KtOutMax=[]  IntegratorOutMin=[]  IntegratorOutMax=[]  FilterOutMin=[]  FilterOutMax=[]  SumI1OutMin=[]  SumI1OutMax=[]  SumI2OutMin=[]  SumI2OutMax=[]  SumI3OutMin=[]  SumI3OutMax=[]  SumI4OutMin=[]  SumI4OutMax=[]  SumDOutMin=[]  SumDOutMax=[]  Sum1OutMin=[]  Sum1OutMax=[]  Sum2OutMin=[]  Sum2OutMax=[]  Sum3OutMin=[]  Sum3OutMax=[]  DifferentiatorOutMin=[]  DifferentiatorOutMax=[]  FilterDiffOutCoefMin=[]  FilterDiffOutCoefMax=[]  ReciprocalOutMin=[]  ReciprocalOutMax=[]  SumDenOutMin=[]  SumDenOutMax=[]  SumNumOutMin=[]  SumNumOutMax=[]  DivideOutMin=[]  DivideOutMax=[]  UdiffTsProdOutMin=[]  UdiffTsProdOutMax=[]  NTsProdOutMin=[]  NTsProdOutMax=[]  UintegralTsProdOutMin=[]  UintegralTsProdOutMax=[]  UngainTsProdOutMin=[]  UngainTsProdOutMax=[]  IntegratorContinuousStateAttributes=''  IntegratorStateMustResolveToSignalObject=off  IntegratorRTWStateStorageClass=Auto  FilterContinuousStateAttributes=''  FilterStateMustResolveToSignalObject=off  FilterRTWStateStorageClass=Auto  ParallelPVariant=InternalParameters  IdealPVariant=Disabled  IVariant=InternalParameters  DVariant=InternalParameters  bVariant=InternalParameters  cVariant=InternalParameters  IntegratorVariant=Discrete  SatVariant=Disabled  AWVariant=Passthrough  PCopyVariant=Disabled  TRVariant=Disabled  FdbkBlocksVariant=Forward  IdealPFdbkVariant=Disabled  SatFdbkVariant=Disabled  DerivativeFilterVariant=ForwardEulerFilter  NVariant=InternalParameters  NCopyVariant=Disabled  FilterICVariant=InternalICsFilter  IntegratorICVariant=InternalICs  ExternalResetVariant=Disabled  TRSumVariant=Passthrough  SumFdbkVariant=Disabled  SumVariant=Sum_PID  TsampFilterVariant=InternalTs  TsampNgainVariant=Passthrough  TsampIntegralVariant=Passthrough  ExternalSaturationOutDataTypeStr=Inherit: Same as second input
      settings: SourceProductBaseCode=SL
  cfblk7 : simulink/Math Operations/MinMax Running Resettable  Function=min  vinit=0.0
  cfblk8 : Sin  TimeSource=Use external signal  SampleTime=0
  cfblk9 : UnaryMinus
  cfblk2 : Outport
  cfblk15 : Outport  Port=2
  wires:
  cfblk10/1 -> cfblk2/1
  cfblk11/1 -> cfblk8/1
  cfblk3/1 -> cfblk15/1
  cfblk12/1 -> cfblk3/1
  cfblk1/1 -> cfblk7/1
  cfblk5/1 -> cfblk9/1
  cfblk4/1 -> cfblk5/1
  cfblk8/1 -> cfblk7/2
  cfblk7/1 -> cfblk6/1
  cfblk14/1 -> cfblk6/2
  cfblk9/1 -> cfblk16/1
  cfblk16/1 -> cfblk4/1

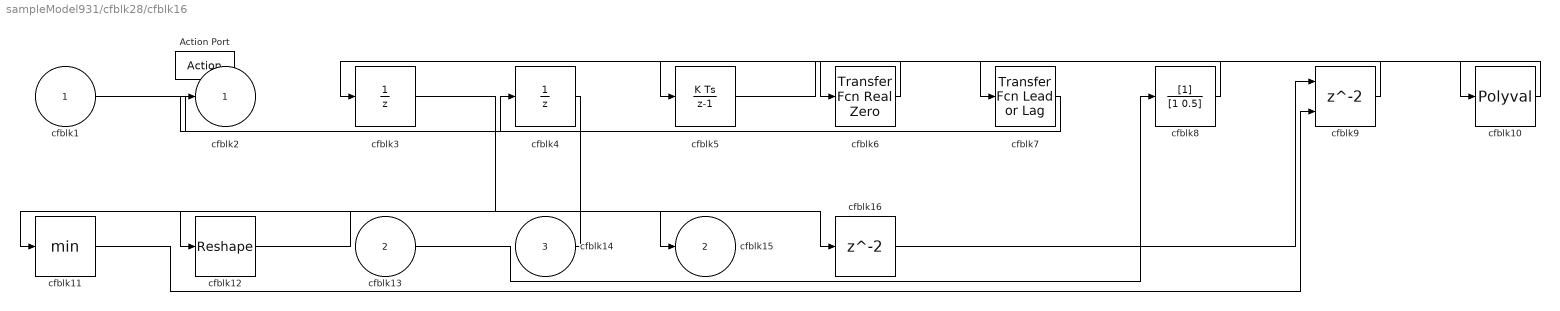
== system sampleModel931/cfblk28/cfblk16 ==
  cfblk1 : Inport
  cfblk13 : Inport  Port=2
  cfblk14 : Inport  Port=3
  Action Port : ActionPort  ActionPortLabel=if(u1 >= 0)
  cfblk10 : Polyval  Coefs=[ +2.081618890e-019, -1.441693666e-014, +4.719686976e-010, -8.536869453e-006, +1.621573104e-001, -8.087801117e+001 ]
  cfblk11 : MinMax
  cfblk12 : Reshape
  cfblk16 : Delay
  cfblk3 : UnitDelay  SampleTime=-1  HasFrameUpgradeWarning=on
  cfblk4 : UnitDelay  SampleTime=-1  HasFrameUpgradeWarning=on
  cfblk5 : DiscreteIntegrator  SampleTime=-1  ICPrevOutput=DiscIntNeverNeededParam  ICPrevScaledInput=DiscIntNeverNeededParam
  cfblk6 : simulink/Discrete/Transfer Fcn Real Zero  ZeroZ=0.75  ICPrevInput=0.0  DoSatur=off
      settings: SourceProductBaseCode=SL
  cfblk7 : simulink/Discrete/Transfer Fcn Lead or Lag  PoleZ=0.95  ZeroZ=0.75  ICPrevOutput=0.0  ICPrevInput=0.0  DoSatur=off
      settings: SourceProductBaseCode=SL
  cfblk8 : DiscreteFilter
  cfblk9 : Delay  ShowEnablePort=on
      settings: InputPortMap=u0,e6
  cfblk2 : Outport
  cfblk15 : Outport  Port=2
  wires:
  cfblk4/1 -> cfblk11/1
  cfblk13/1 -> cfblk8/1
  cfblk1/1 -> cfblk4/1
  cfblk12/1 -> cfblk15/1
  cfblk6/1 -> cfblk3/1
  cfblk8/1 -> cfblk5/1
  cfblk14/1 -> cfblk12/1
  cfblk10/1 -> cfblk7/1
  cfblk11/1 -> cfblk9/2
  cfblk9/1 -> cfblk6/1
  cfblk5/1 -> cfblk10/1
  cfblk7/1 -> cfblk2/1
  cfblk3/1 -> cfblk16/1
  cfblk16/1 -> cfblk9/1

== system sampleModel931/cfblk28/cfblk17 ==
  cfblk1 : Inport
  cfblk11 : Inport  Port=2
  cfblk12 : Inport  Port=3
  Action Port : ActionPort  ActionPortLabel=else
  cfblk10 : Sum  Inputs=+
  cfblk15 : Delay
  cfblk3 : Delay
  cfblk4 : DiscreteFilter
  cfblk5 : simulink/Discrete/Transfer Fcn Real Zero  ZeroZ=0.75  ICPrevInput=0.0  DoSatur=off
      settings: SourceProductBaseCode=SL
  cfblk6 : DiscreteZeroPole  Poles=[0 0.5]  Gain=1  SampleTime=-1
  cfblk7 : simulink/Discrete/Transfer Fcn Real Zero  ZeroZ=0.75  ICPrevInput=0.0  DoSatur=off
      settings: SourceProductBaseCode=SL
  cfblk8 : Sum  Inputs=|++
  cfblk9 : Sum  Inputs=+-
  cfblk2 : Outport
  cfblk13 : Outport  Port=2
  cfblk14 : Outport  Port=3
  wires:
  cfblk12/1 -> cfblk5/1
  cfblk5/1 -> cfblk4/1
  cfblk3/1 -> cfblk10/1
  cfblk10/1 -> cfblk9/1
  cfblk6/1 -> cfblk13/1, cfblk8/1, cfblk8/2
  cfblk1/1 -> cfblk3/1
  cfblk4/1 -> cfblk2/1
  cfblk9/1 -> cfblk7/1
  cfblk11/1 -> cfblk9/2
  cfblk7/1 -> cfblk14/1
  cfblk8/1 -> cfblk15/1
  cfblk15/1 -> cfblk6/1

== system sampleModel931/cfblk28/cfblk7 ==
  cfblk1 : Inport
  cfblk10 : Inport  Port=2
  cfblk11 : Inport  Port=3
  cfblk12 : Inport  Port=4
  cfblk13 : Inport  Port=5
  cfblk15 : Delay  SampleTime=1
  cfblk3 : pid_lib/PID Controller (2DOF)  Controller=PID  Form=Parallel  TimeDomain=Discrete-time  UseExternalTs=off  SampleTime=1  IntegratorMethod=Forward Euler  FilterMethod=Forward Euler  ControllerParametersSource=internal  P=1  I=1  D=0  UseFilter=on  N=100  b=1  c=1  TunerSelectOption=Transfer Function Based (PID Tuner App)  InitialConditionSource=internal  InitialConditionForIntegrator=0  InitialConditionForFilter=0  DifferentiatorICPrevScaledInput=0  ExternalReset=none  TrackingMode=off  Kt=1  LimitOutput=off  SatLimitsSource=internal  UpperSaturationLimit=inf  LowerSaturationLimit=-inf  LinearizeAsGain=off  AntiWindupMode=none  Kb=1  POutMin=[]  POutMax=[]  IOutMin=[]  IOutMax=[]  DOutMin=[]  DOutMax=[]  NOutMin=[]  NOutMax=[]  bOutMin=[]  bOutMax=[]  cOutMin=[]  cOutMax=[]  SumOutMin=[]  SumOutMax=[]  SaturationOutMin=[]  SaturationOutMax=[]  PParamMin=[]  PParamMax=[]  IParamMin=[]  IParamMax=[]  DParamMin=[]  DParamMax=[]  NParamMin=[]  NParamMax=[]  bParamMin=[]  bParamMax=[]  cParamMin=[]  cParamMax=[]  KbParamMin=[]  KbParamMax=[]  KtParamMin=[]  KtParamMax=[]  KbOutMin=[]  KbOutMax=[]  KtOutMin=[]  KtOutMax=[]  IntegratorOutMin=[]  IntegratorOutMax=[]  FilterOutMin=[]  FilterOutMax=[]  SumI1OutMin=[]  SumI1OutMax=[]  SumI2OutMin=[]  SumI2OutMax=[]  SumI3OutMin=[]  SumI3OutMax=[]  SumI4OutMin=[]  SumI4OutMax=[]  SumDOutMin=[]  SumDOutMax=[]  Sum1OutMin=[]  Sum1OutMax=[]  Sum2OutMin=[]  Sum2OutMax=[]  Sum3OutMin=[]  Sum3OutMax=[]  DifferentiatorOutMin=[]  DifferentiatorOutMax=[]  FilterDiffOutCoefMin=[]  FilterDiffOutCoefMax=[]  ReciprocalOutMin=[]  ReciprocalOutMax=[]  SumDenOutMin=[]  SumDenOutMax=[]  SumNumOutMin=[]  SumNumOutMax=[]  DivideOutMin=[]  DivideOutMax=[]  UdiffTsProdOutMin=[]  UdiffTsProdOutMax=[]  NTsProdOutMin=[]  NTsProdOutMax=[]  UintegralTsProdOutMin=[]  UintegralTsProdOutMax=[]  UngainTsProdOutMin=[]  UngainTsProdOutMax=[]  IntegratorContinuousStateAttributes=''  IntegratorStateMustResolveToSignalObject=off  IntegratorRTWStateStorageClass=Auto  FilterContinuousStateAttributes=''  FilterStateMustResolveToSignalObject=off  FilterRTWStateStorageClass=Auto  ParallelPVariant=InternalParameters  IdealPVariant=Disabled  IVariant=InternalParameters  DVariant=InternalParameters  bVariant=InternalParameters  cVariant=InternalParameters  IntegratorVariant=Discrete  SatVariant=Disabled  AWVariant=Passthrough  PCopyVariant=Disabled  TRVariant=Disabled  FdbkBlocksVariant=Forward  IdealPFdbkVariant=Disabled  SatFdbkVariant=Disabled  DerivativeFilterVariant=ForwardEulerFilter  NVariant=InternalParameters  NCopyVariant=Disabled  FilterICVariant=InternalICsFilter  IntegratorICVariant=InternalICs  ExternalResetVariant=Disabled  TRSumVariant=Passthrough  SumFdbkVariant=Disabled  SumVariant=Sum_PID  TsampFilterVariant=InternalTs  TsampNgainVariant=Passthrough  TsampIntegralVariant=Passthrough  ExternalSaturationOutDataTypeStr=Inherit: Same as second input
      settings: SourceProductBaseCode=SL
  cfblk4 : DiscreteFir  SampleTime=1
  cfblk5 : MinMax  Function=max  Inputs=3
  cfblk6 : Abs
  cfblk7 : Sum  Inputs=--
  cfblk8 : PermuteDimensions
  cfblk9 : simulink/Math Operations/Slider Gain  gain=1  low=0  high=2
  cfblk2 : Outport
  cfblk14 : Outport  Port=2
  wires:
  cfblk11/1 -> cfblk5/1
  cfblk12/1 -> cfblk5/2, cfblk7/2
  cfblk13/1 -> cfblk5/3
  cfblk3/1 -> cfblk8/1
  cfblk5/1 -> cfblk4/1
  cfblk8/1 -> cfblk6/1
  cfblk9/1 -> cfblk2/1
  cfblk10/1 -> cfblk14/1
  cfblk4/1 -> cfblk3/2
  cfblk7/1 -> cfblk9/1
  cfblk1/1 -> cfblk7/1
  cfblk6/1 -> cfblk15/1
  cfblk15/1 -> cfblk3/1

== system sampleModel931/cfblk28/cfblk8 ==
  cfblk1 : Inport
  cfblk3 : Squeeze
  cfblk4 : Sin  TimeSource=Use external signal  SampleTime=0
  cfblk5 : Sum  Inputs=+
  cfblk6 : ComplexToRealImag
  cfblk7 : Sum  Inputs=|++
  cfblk9 : Delay  SampleTime=1
  cfblk2 : Outport
  cfblk8 : Outport  Port=2
  wires:
  cfblk6/1 -> cfblk4/1
  cfblk1/1 -> cfblk3/1
  cfblk5/1 -> cfblk6/1
  cfblk3/1 -> cfblk7/1
  cfblk6/2 -> cfblk8/1, cfblk9/1
  cfblk7/1 -> cfblk5/1
  cfblk4/1 -> cfblk2/1
  cfblk9/1 -> cfblk7/2

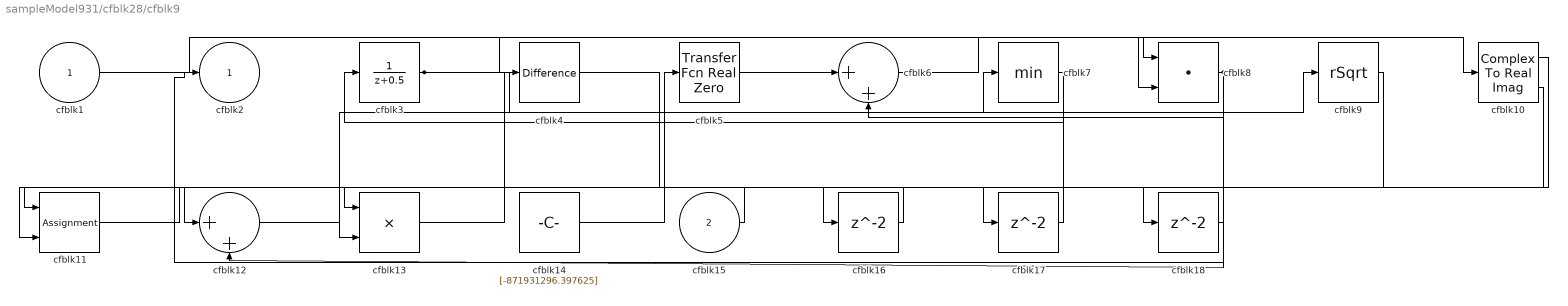
== system sampleModel931/cfblk28/cfblk9 ==
  cfblk1 : Inport
  cfblk15 : Inport  Port=2
  cfblk10 : ComplexToRealImag
  cfblk11 : Assignment  DiagnosticForDimensions=Warning  IndexOptions=Index vector (dialog)  Indices=1  OutputSizes=1
  cfblk12 : Sum  Inputs=|++
  cfblk13 : Product
  cfblk14 : Constant  Value=[-871931296.397625]  SampleTime=1
  cfblk16 : Delay  SampleTime=1
  cfblk17 : Delay  SampleTime=1
  cfblk18 : Delay  SampleTime=1
  cfblk3 : DiscreteTransferFcn  SampleTime=1
  cfblk4 : simulink/Discrete/Difference  ICPrevInput=0.0  OutMin=[]  OutMax=[]  OutDataTypeStr=Inherit: Inherit via back propagation  OutDataType=fixdt(1, 16)  OutScaling=2^-10  DoSatur=off
  cfblk5 : simulink/Discrete/Transfer Fcn Real Zero  ZeroZ=0.75  ICPrevInput=0.0  DoSatur=off
      settings: SourceProductBaseCode=SL
  cfblk6 : Sum  Inputs=|++
  cfblk7 : MinMax
  cfblk8 : DotProduct  InputSameDT=on  OutDataTypeStr=Inherit: Inherit via internal rule
  cfblk9 : Sqrt  Operator=rSqrt  AlgorithmType=Newton-Raphson  SaturateOnIntegerOverflow=on
  cfblk2 : Outport
  wires:
  cfblk3/1 -> cfblk7/1, cfblk8/2
  cfblk6/1 -> cfblk10/1
  cfblk14/1 -> cfblk5/1
  cfblk1/1 -> cfblk8/1
  cfblk13/1 -> cfblk4/1
  cfblk8/1 -> cfblk2/1, cfblk12/2
  cfblk10/1 -> cfblk13/1
  cfblk5/1 -> cfblk6/1
  cfblk12/1 -> cfblk9/1
  cfblk9/1 -> cfblk13/2
  cfblk15/1 -> cfblk11/1
  cfblk10/2 -> cfblk11/2
  cfblk4/1 -> cfblk16/1
  cfblk16/1 -> cfblk12/1
  cfblk7/1 -> cfblk17/1
  cfblk17/1 -> cfblk3/1
  cfblk11/1 -> cfblk18/1
  cfblk18/1 -> cfblk6/2

== system sampleModel931/cfblk29/cfblk10 ==
  cfblk1 : Inport
  cfblk6 : Inport  Port=2
  cfblk7 : Inport  Port=3
  cfblk8 : Inport  Port=4
  cfblk11 : Delay  SampleTime=1
  cfblk3 : Sum  Inputs=|++
  cfblk4 : Sqrt  SaturateOnIntegerOverflow=on
  cfblk5 : Sqrt  Operator=rSqrt  AlgorithmType=Newton-Raphson  SaturateOnIntegerOverflow=on
  cfblk2 : Outport
  cfblk9 : Outport  Port=2
  cfblk10 : Outport  Port=3
  wires:
  cfblk6/1 -> cfblk9/1
  cfblk8/1 -> cfblk4/1
  cfblk1/1 -> cfblk3/1
  cfblk4/1 -> cfblk10/1
  cfblk7/1 -> cfblk2/1
  cfblk3/1 -> cfblk5/1
  cfblk5/1 -> cfblk11/1
  cfblk11/1 -> cfblk3/2

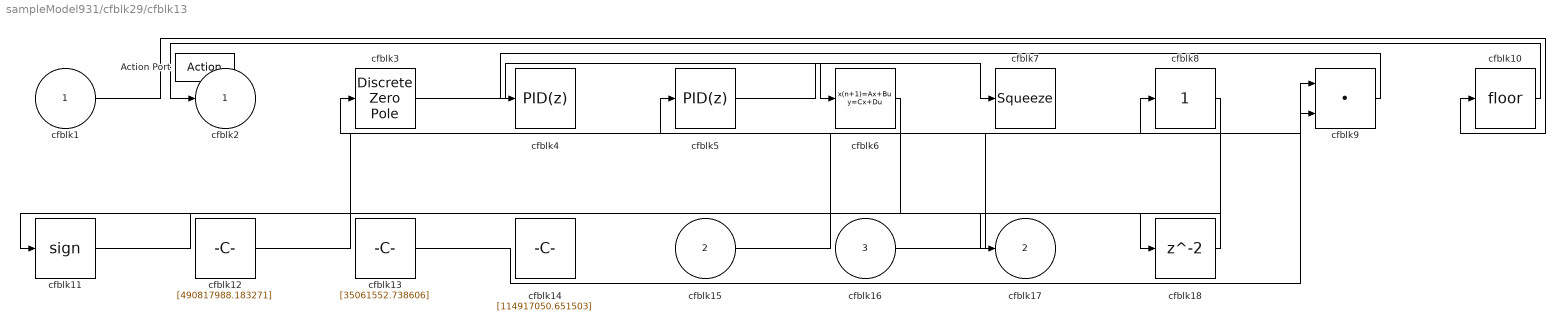
== system sampleModel931/cfblk29/cfblk13 ==
  cfblk1 : Inport
  cfblk15 : Inport  Port=2
  cfblk16 : Inport  Port=3
  Action Port : ActionPort  ActionPortLabel=if(u1 >= 0)
  cfblk10 : Rounding
  cfblk11 : Signum
  cfblk12 : Constant  Value=[490817988.183271]  SampleTime=1
  cfblk13 : Constant  Value=[35061552.738606]  SampleTime=1
  cfblk14 : Constant  Value=[114917050.651503]  SampleTime=1
  cfblk18 : Delay
  cfblk3 : DiscreteZeroPole  Poles=[0 0.5]  Gain=1  SampleTime=-1
  cfblk4 : pid_lib/PID Controller  Controller=PID  Form=Parallel  TimeDomain=Discrete-time  UseExternalTs=off  SampleTime=-1  IntegratorMethod=Forward Euler  FilterMethod=Forward Euler  ControllerParametersSource=internal  P=1  I=1  D=0  UseFilter=on  N=100  TunerSelectOption=Transfer Function Based (PID Tuner App)  InitialConditionSource=internal  InitialConditionForIntegrator=0  InitialConditionForFilter=0  DifferentiatorICPrevScaledInput=0  ExternalReset=none  TrackingMode=off  Kt=1  LimitOutput=off  SatLimitsSource=internal  UpperSaturationLimit=inf  LowerSaturationLimit=-inf  LinearizeAsGain=off  AntiWindupMode=none  Kb=1  POutMin=[]  POutMax=[]  IOutMin=[]  IOutMax=[]  DOutMin=[]  DOutMax=[]  NOutMin=[]  NOutMax=[]  SumOutMin=[]  SumOutMax=[]  SaturationOutMin=[]  SaturationOutMax=[]  PParamMin=[]  PParamMax=[]  IParamMin=[]  IParamMax=[]  DParamMin=[]  DParamMax=[]  NParamMin=[]  NParamMax=[]  KbParamMin=[]  KbParamMax=[]  KtParamMin=[]  KtParamMax=[]  KbOutMin=[]  KbOutMax=[]  KtOutMin=[]  KtOutMax=[]  IntegratorOutMin=[]  IntegratorOutMax=[]  FilterOutMin=[]  FilterOutMax=[]  SumI1OutMin=[]  SumI1OutMax=[]  SumI2OutMin=[]  SumI2OutMax=[]  SumI3OutMin=[]  SumI3OutMax=[]  SumI4OutMin=[]  SumI4OutMax=[]  SumDOutMin=[]  SumDOutMax=[]  DifferentiatorOutMin=[]  DifferentiatorOutMax=[]  FilterDiffOutCoefMin=[]  FilterDiffOutCoefMax=[]  ReciprocalOutMin=[]  ReciprocalOutMax=[]  SumDenOutMin=[]  SumDenOutMax=[]  SumNumOutMin=[]  SumNumOutMax=[]  DivideOutMin=[]  DivideOutMax=[]  UdiffTsProdOutMin=[]  UdiffTsProdOutMax=[]  NTsProdOutMin=[]  NTsProdOutMax=[]  UintegralTsProdOutMin=[]  UintegralTsProdOutMax=[]  UngainTsProdOutMin=[]  UngainTsProdOutMax=[]  IntegratorContinuousStateAttributes=''  IntegratorStateMustResolveToSignalObject=off  IntegratorRTWStateStorageClass=Auto  FilterContinuousStateAttributes=''  FilterStateMustResolveToSignalObject=off  FilterRTWStateStorageClass=Auto  ParallelPVariant=InternalParameters  IdealPVariant=Disabled  IVariant=InternalParameters  DVariant=InternalParameters  IntegratorVariant=Discrete  SatVariant=Disabled  AWVariant=Passthrough  PCopyVariant=Disabled  TRVariant=Disabled  FdbkBlocksVariant=Forward  IdealPFdbkVariant=Disabled  SatFdbkVariant=Disabled  DerivativeFilterVariant=ForwardEulerFilter  NVariant=InternalParameters  NCopyVariant=Disabled  FilterICVariant=InternalICsFilter  IntegratorICVariant=InternalICs  ExternalResetVariant=Disabled  TRSumVariant=Passthrough  SumFdbkVariant=Disabled  SumVariant=Sum_PID  TsampFilterVariant=InternalTs  TsampNgainVariant=Passthrough  TsampIntegralVariant=Passthrough  ExternalSaturationOutDataTypeStr=Inherit: Same as second input
  cfblk5 : pid_lib/PID Controller  Controller=PID  Form=Parallel  TimeDomain=Discrete-time  UseExternalTs=off  SampleTime=-1  IntegratorMethod=Forward Euler  FilterMethod=Forward Euler  ControllerParametersSource=internal  P=1  I=1  D=0  UseFilter=on  N=100  TunerSelectOption=Transfer Function Based (PID Tuner App)  InitialConditionSource=internal  InitialConditionForIntegrator=0  InitialConditionForFilter=0  DifferentiatorICPrevScaledInput=0  ExternalReset=none  TrackingMode=off  Kt=1  LimitOutput=off  SatLimitsSource=internal  UpperSaturationLimit=inf  LowerSaturationLimit=-inf  LinearizeAsGain=off  AntiWindupMode=none  Kb=1  POutMin=[]  POutMax=[]  IOutMin=[]  IOutMax=[]  DOutMin=[]  DOutMax=[]  NOutMin=[]  NOutMax=[]  SumOutMin=[]  SumOutMax=[]  SaturationOutMin=[]  SaturationOutMax=[]  PParamMin=[]  PParamMax=[]  IParamMin=[]  IParamMax=[]  DParamMin=[]  DParamMax=[]  NParamMin=[]  NParamMax=[]  KbParamMin=[]  KbParamMax=[]  KtParamMin=[]  KtParamMax=[]  KbOutMin=[]  KbOutMax=[]  KtOutMin=[]  KtOutMax=[]  IntegratorOutMin=[]  IntegratorOutMax=[]  FilterOutMin=[]  FilterOutMax=[]  SumI1OutMin=[]  SumI1OutMax=[]  SumI2OutMin=[]  SumI2OutMax=[]  SumI3OutMin=[]  SumI3OutMax=[]  SumI4OutMin=[]  SumI4OutMax=[]  SumDOutMin=[]  SumDOutMax=[]  DifferentiatorOutMin=[]  DifferentiatorOutMax=[]  FilterDiffOutCoefMin=[]  FilterDiffOutCoefMax=[]  ReciprocalOutMin=[]  ReciprocalOutMax=[]  SumDenOutMin=[]  SumDenOutMax=[]  SumNumOutMin=[]  SumNumOutMax=[]  DivideOutMin=[]  DivideOutMax=[]  UdiffTsProdOutMin=[]  UdiffTsProdOutMax=[]  NTsProdOutMin=[]  NTsProdOutMax=[]  UintegralTsProdOutMin=[]  UintegralTsProdOutMax=[]  UngainTsProdOutMin=[]  UngainTsProdOutMax=[]  IntegratorContinuousStateAttributes=''  IntegratorStateMustResolveToSignalObject=off  IntegratorRTWStateStorageClass=Auto  FilterContinuousStateAttributes=''  FilterStateMustResolveToSignalObject=off  FilterRTWStateStorageClass=Auto  ParallelPVariant=InternalParameters  IdealPVariant=Disabled  IVariant=InternalParameters  DVariant=InternalParameters  IntegratorVariant=Discrete  SatVariant=Disabled  AWVariant=Passthrough  PCopyVariant=Disabled  TRVariant=Disabled  FdbkBlocksVariant=Forward  IdealPFdbkVariant=Disabled  SatFdbkVariant=Disabled  DerivativeFilterVariant=ForwardEulerFilter  NVariant=InternalParameters  NCopyVariant=Disabled  FilterICVariant=InternalICsFilter  IntegratorICVariant=InternalICs  ExternalResetVariant=Disabled  TRSumVariant=Passthrough  SumFdbkVariant=Disabled  SumVariant=Sum_PID  TsampFilterVariant=InternalTs  TsampNgainVariant=Passthrough  TsampIntegralVariant=Passthrough  ExternalSaturationOutDataTypeStr=Inherit: Same as second input
  cfblk6 : DiscreteStateSpace  SampleTime=-1
  cfblk7 : Squeeze
  cfblk8 : simulink/Math Operations/Slider Gain  gain=1  low=0  high=2
  cfblk9 : DotProduct  InputSameDT=on  OutDataTypeStr=Inherit: Inherit via internal rule
  cfblk2 : Outport
  cfblk17 : Outport  Port=2
  wires:
  cfblk3/1 -> cfblk6/1
  cfblk6/1 -> cfblk11/1
  cfblk5/1 -> cfblk7/1
  cfblk9/1 -> cfblk4/1
  cfblk16/1 -> cfblk8/1
  cfblk10/1 -> cfblk2/1
  cfblk13/1 -> cfblk9/1
  cfblk15/1 -> cfblk9/2
  cfblk1/1 -> cfblk10/1
  cfblk12/1 -> cfblk5/1
  cfblk8/1 -> cfblk17/1
  cfblk11/1 -> cfblk18/1
  cfblk18/1 -> cfblk3/1

== system sampleModel931/cfblk29/cfblk14 ==
  cfblk1 : Inport
  cfblk12 : Inport  Port=2
  cfblk13 : Inport  Port=3
  cfblk14 : Inport  Port=4
  Action Port : ActionPort  ActionPortLabel=else
  cfblk10 : Sin  TimeSource=Use external signal  SampleTime=0
  cfblk11 : Constant  Value=[230499246.727005]  SampleTime=1
  cfblk3 : DiscreteFilter
  cfblk4 : Polyval  Coefs=[ +2.081618890e-019, -1.441693666e-014, +4.719686976e-010, -8.536869453e-006, +1.621573104e-001, -8.087801117e+001 ]
  cfblk5 : Assignment  DiagnosticForDimensions=Warning  IndexOptions=Index vector (dialog)  Indices=1  OutputSizes=1
  cfblk6 : Sin  TimeSource=Use external signal  SampleTime=0
  cfblk7 : Assignment  DiagnosticForDimensions=Warning  IndexOptions=Index vector (dialog)  Indices=1  OutputSizes=1
  cfblk8 : Trigonometry
  cfblk9 : Assignment  DiagnosticForDimensions=Warning  IndexOptions=Index vector (dialog)  Indices=1  OutputSizes=1
  cfblk2 : Outport
  wires:
  cfblk7/1 -> cfblk2/1
  cfblk5/1 -> cfblk6/1
  cfblk4/1 -> cfblk10/1
  cfblk14/1 -> cfblk8/1
  cfblk3/1 -> cfblk4/1
  cfblk8/1 -> cfblk7/1
  cfblk6/1 -> cfblk9/1
  cfblk11/1 -> cfblk9/2
  cfblk10/1 -> cfblk7/2
  cfblk9/1 -> cfblk3/1
  cfblk1/1 -> cfblk5/1
  cfblk12/1 -> cfblk5/2

== system sampleModel931/cfblk29/cfblk9 ==
  cfblk1 : Inport
  cfblk8 : Inport  Port=2
  cfblk3 : simulink/Discrete/Tapped Delay  vinit=0.0  samptime=-1  NumDelays=1  DelayOrder=Oldest  includeCurrent=off
  cfblk4 : Squeeze
  cfblk5 : Sin  TimeSource=Use external signal  SampleTime=0
  cfblk6 : Reshape
  cfblk7 : Product
  cfblk2 : Outport
  wires:
  cfblk6/1 -> cfblk4/1
  cfblk7/1 -> cfblk2/1
  cfblk8/1 -> cfblk7/1
  cfblk1/1 -> cfblk5/1
  cfblk5/1 -> cfblk6/1
  cfblk4/1 -> cfblk3/1
  cfblk3/1 -> cfblk7/2

== system sampleModel931/cfblk31/cfblk11 ==
  cfblk1 : Inport
  cfblk6 : Inport  Port=2
  cfblk3 : UnitDelay  HasFrameUpgradeWarning=on
  cfblk4 : simulink/Discrete/Difference  ICPrevInput=0.0  OutMin=[]  OutMax=[]  OutDataTypeStr=Inherit: Inherit via back propagation  OutDataType=fixdt(1, 16)  OutScaling=2^-10  DoSatur=off
  cfblk5 : Sum  Inputs=--
  cfblk2 : Outport
  cfblk7 : Outport  Port=2
  wires:
  cfblk5/1 -> cfblk7/1
  cfblk6/1 -> cfblk2/1
  cfblk1/1 -> cfblk3/1
  cfblk3/1 -> cfblk4/1, cfblk5/2
  cfblk4/1 -> cfblk5/1

== system sampleModel931/cfblk31/cfblk12 ==
  cfblk1 : Inport
  cfblk10 : Inport  Port=2
  cfblk11 : Inport  Port=3
  cfblk3 : Delay  ShowEnablePort=on  SampleTime=1
      settings: InputPortMap=u0,e6
  cfblk4 : Delay  ShowEnablePort=on  SampleTime=1
      settings: InputPortMap=u0,e6
  cfblk5 : simulink/Math Operations/Slider Gain  gain=1  low=0  high=2
  cfblk6 : Product  Inputs=*
  cfblk7 : Constant  Value=[928871332.694169]  SampleTime=1
  cfblk8 : Constant  Value=[880176890.051902]  SampleTime=1
  cfblk9 : Constant  Value=[632141078.379802]  SampleTime=1
  cfblk2 : Outport
  cfblk12 : Outport  Port=2
  cfblk13 : Outport  Port=3
  cfblk14 : Outport  Port=4
  wires:
  cfblk1/1 -> cfblk3/1
  cfblk8/1 -> cfblk14/1
  cfblk11/1 -> cfblk13/1
  cfblk9/1 -> cfblk12/1
  cfblk5/1 -> cfblk3/2
  cfblk4/1 -> cfblk6/1
  cfblk3/1 -> cfblk2/1
  cfblk6/1 -> cfblk5/1
  cfblk7/1 -> cfblk4/1
  cfblk10/1 -> cfblk4/2

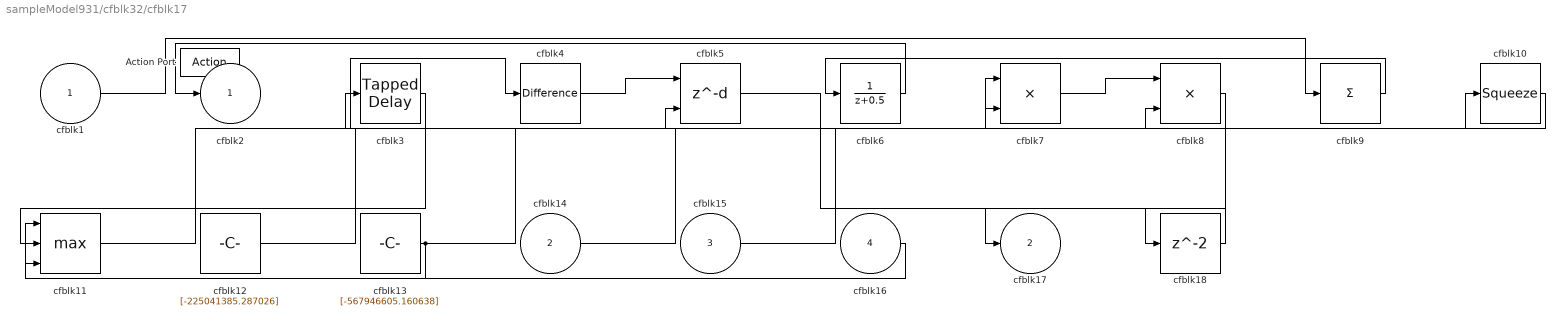
== system sampleModel931/cfblk32/cfblk17 ==
  cfblk1 : Inport
  cfblk14 : Inport  Port=2
  cfblk15 : Inport  Port=3
  cfblk16 : Inport  Port=4
  Action Port : ActionPort  ActionPortLabel=if(u1 >= 0)
  cfblk10 : Squeeze
  cfblk11 : MinMax  Function=max  Inputs=3
  cfblk12 : Constant  Value=[-225041385.287026]  SampleTime=1
  cfblk13 : Constant  Value=[-567946605.160638]  SampleTime=1
  cfblk18 : Delay
  cfblk3 : simulink/Discrete/Tapped Delay  vinit=0.0  samptime=-1  NumDelays=1  DelayOrder=Oldest  includeCurrent=off
  cfblk4 : simulink/Discrete/Difference  ICPrevInput=0.0  OutMin=[]  OutMax=[]  OutDataTypeStr=Inherit: Inherit via back propagation  OutDataType=fixdt(1, 16)  OutScaling=2^-10  DoSatur=off
  cfblk5 : Delay  DelayLengthSource=Input port
      settings: InputPortMap=u0,p1
  cfblk6 : DiscreteTransferFcn
  cfblk7 : Product  Inputs=**
  cfblk8 : Product  Inputs=**
  cfblk9 : Sum  Inputs=+
  cfblk2 : Outport
  cfblk17 : Outport  Port=2
  wires:
  cfblk12/1 -> cfblk10/1
  cfblk4/1 -> cfblk5/1
  cfblk10/1 -> cfblk5/2
  cfblk6/1 -> cfblk2/1
  cfblk1/1 -> cfblk9/1
  cfblk11/1 -> cfblk4/1
  cfblk16/1 -> cfblk11/1
  cfblk15/1 -> cfblk7/1
  cfblk3/1 -> cfblk11/2
  cfblk8/1 -> cfblk17/1
  cfblk14/1 -> cfblk7/2
  cfblk9/1 -> cfblk6/1
  cfblk7/1 -> cfblk8/1
  cfblk13/1 -> cfblk8/2, cfblk11/3
  cfblk5/1 -> cfblk18/1
  cfblk18/1 -> cfblk3/1

== system sampleModel931/cfblk32/cfblk18 ==
  cfblk1 : Inport
  cfblk9 : Inport  Port=2
  cfblk10 : Inport  Port=3
  Action Port : ActionPort  ActionPortLabel=else
  cfblk3 : DiscreteFir
  cfblk4 : Abs
  cfblk5 : Assignment  DiagnosticForDimensions=Warning  IndexOptions=Index vector (dialog)  Indices=1  OutputSizes=1
  cfblk6 : Product  Inputs=**
  cfblk7 : Constant  Value=[-35498714.014685]  SampleTime=1
  cfblk8 : Constant  Value=[194252932.701550]  SampleTime=1
  cfblk2 : Outport
  cfblk11 : Outport  Port=2
  cfblk12 : Outport  Port=3
  wires:
  cfblk8/1 -> cfblk2/1
  cfblk9/1 -> cfblk6/1
  cfblk1/1 -> cfblk6/2
  cfblk5/1 -> cfblk12/1
  cfblk4/1 -> cfblk11/1
  cfblk7/1 -> cfblk5/1
  cfblk3/1 -> cfblk4/1
  cfblk10/1 -> cfblk5/2
  cfblk6/1 -> cfblk3/1

== system sampleModel931/cfblk33/cfblk10 ==
  cfblk1 : Inport
  cfblk7 : Inport  Port=2
  cfblk8 : Inport  Port=3
  cfblk3 : Delay  ShowEnablePort=on  SampleTime=1
      settings: InputPortMap=u0,e6
  cfblk4 : DiscreteFir  SampleTime=1
  cfblk5 : DiscreteFir  SampleTime=1
  cfblk6 : ComplexToMagnitudeAngle
  cfblk2 : Outport
  cfblk9 : Outport  Port=2
  wires:
  cfblk6/1 -> cfblk4/1
  cfblk6/2 -> cfblk9/1
  cfblk1/1 -> cfblk5/1
  cfblk4/1 -> cfblk2/1
  cfblk5/1 -> cfblk3/1
  cfblk8/1 -> cfblk3/2
  cfblk7/1 -> cfblk6/1
